simulink model "pendulum_balance"  (R2022a)
settings: Solver=VariableStepAuto  StartTime=0.0  StopTime=10.0  RelTol=1e-3
settings Model: Creator=anthony  LastModifiedBy=anthony

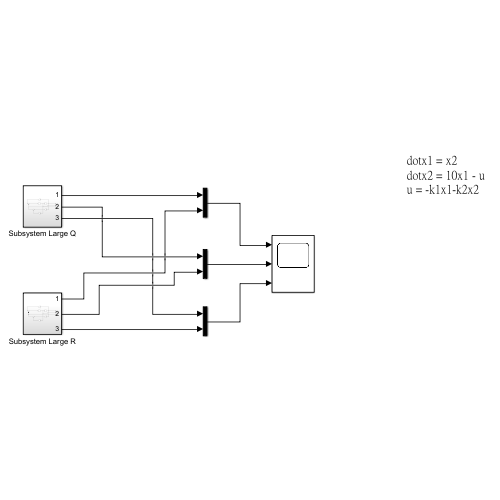
[thumbnail: Simulink's stored preview of the top-level diagram]
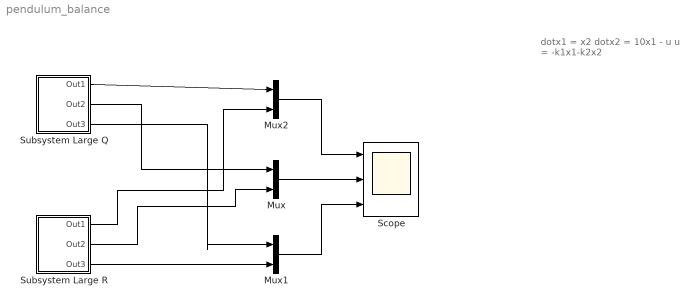
== system pendulum_balance ==
  note: dotx1 = x2
      | dotx2 = 10x1 - u
      | u = -k1x1-k2x2
  Mux : Mux  Inputs=2
  Mux1 : Mux  Inputs=2
  Mux2 : Mux  Inputs=2
  Scope : Scope  NumInputPorts=3
  Subsystem Large Q : Subsystem
  Subsystem Large R : Subsystem
  wires:
  Subsystem Large Q/1(Out1) -> Mux2/1
  Subsystem Large Q/2(Out2) -> Mux/1
  Subsystem Large Q/3(Out3) -> Mux1/1
  Subsystem Large R/1(Out1) -> Mux2/2
  Subsystem Large R/2(Out2) -> Mux/2
  Subsystem Large R/3(Out3) -> Mux1/2
  Mux/1 -> Scope/2
  Mux2/1 -> Scope/1
  Mux1/1 -> Scope/3

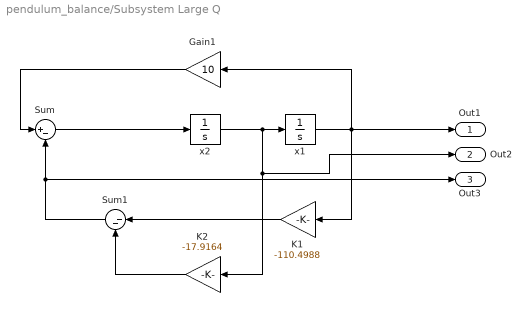
== system pendulum_balance/Subsystem Large Q ==
  Gain1 : Gain  Gain=10
  K1 : Gain  Gain=-110.4988
  K2 : Gain  Gain=-17.9164
  Sum : Sum  Inputs=|+-
  Sum1 : Sum  Inputs=|--
  x1 : Integrator  InitialCondition=5
  x2 : Integrator
  Out1 : Outport
  Out2 : Outport  Port=2
  Out3 : Outport  Port=3
  wires:
  Sum/1 -> x2/1
  Gain1/1 -> Sum/1
  Sum1/1 -> Out3/1, Sum/2
  x2/1 -> Out2/1, K2/1, x1/1
  K1/1 -> Sum1/1
  x1/1 -> Out1/1, Gain1/1, K1/1
  K2/1 -> Sum1/2

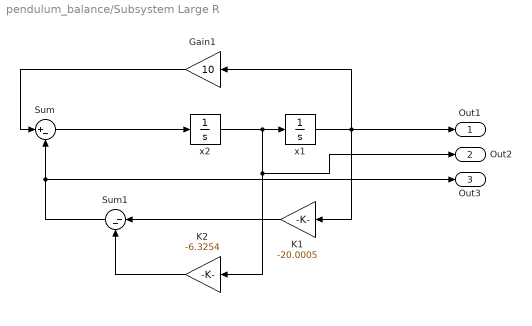
== system pendulum_balance/Subsystem Large R ==
  Gain1 : Gain  Gain=10
  K1 : Gain  Gain=-20.0005
  K2 : Gain  Gain=-6.3254
  Sum : Sum  Inputs=|+-
  Sum1 : Sum  Inputs=|--
  x1 : Integrator  InitialCondition=5
  x2 : Integrator
  Out1 : Outport
  Out2 : Outport  Port=2
  Out3 : Outport  Port=3
  wires:
  K2/1 -> Sum1/2
  x1/1 -> K1/1, Gain1/1, Out1/1
  K1/1 -> Sum1/1
  x2/1 -> x1/1, K2/1, Out2/1
  Sum1/1 -> Sum/2, Out3/1
  Gain1/1 -> Sum/1
  Sum/1 -> x2/1
